simulink model "relative_dynamics_Earth_SK"  (R2021a)
settings: Solver=VariableStepAuto  StartTime=0.0  StopTime=53020  FixedStep=5  RelTol=1e-9  AbsTol=1e-11
undefined symbols (not defined in the file): a, d_lp, d_lp_sk, d_lp_z, e, init_conds, init_conds_z, K, K_z, km, M, M_z, n, n_lp, n_lp_sk, n_lp_z, r_target, s
libraries: vrlib x3, aerolibcelestial x2
settings Model: Creator=danie  LastModifiedBy=danie
settings SolverCC: AlgebraicLoopSolver=TrustRegion
settings DebuggingCC: SFMachineParentedDataDiag=warning

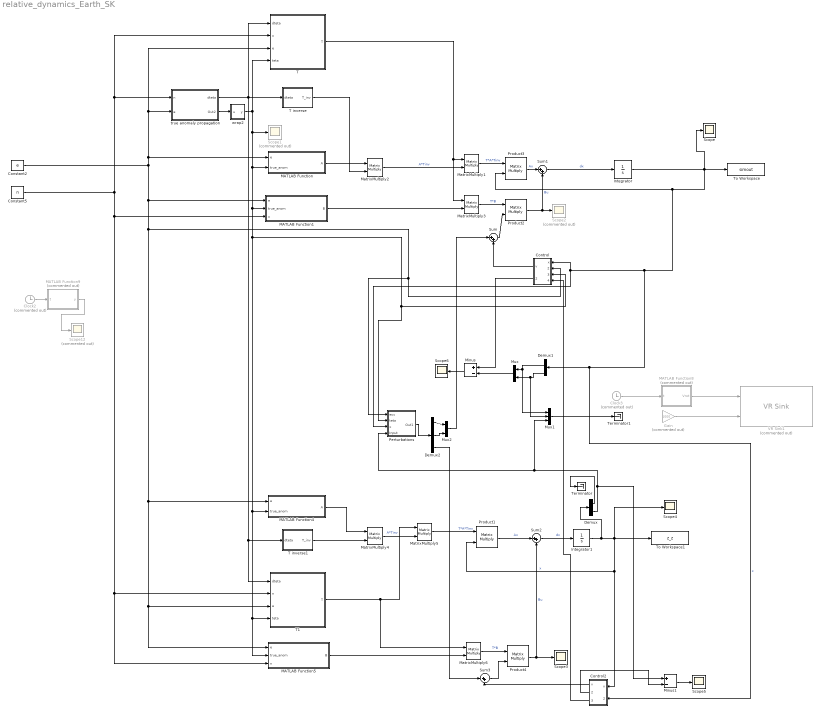
== system relative_dynamics_Earth_SK ==
  Clock2 : Clock  Commented=on
  Clock3 : Clock  Commented=on
  Constant2 : Constant  Value=e
  Constant5 : Constant  Value=n
  Control : Subsystem
  Control2 : Subsystem
  Demux : Demux  Outputs=2
  Demux1 : Demux
  Demux2 : Demux  Outputs=3
  Gain : Gain  Commented=on  Gain=1000
  Integrator : Integrator  InitialCondition=init_conds
  Integrator1 : Integrator  InitialCondition=init_conds_z
  MATLAB Function : MATLAB Function  TreatAsAtomicUnit=on
  MATLAB Function1 : MATLAB Function  TreatAsAtomicUnit=on
  MATLAB Function4 : MATLAB Function  TreatAsAtomicUnit=on
  MATLAB Function5 : MATLAB Function  TreatAsAtomicUnit=on
  MATLAB Function8 : MATLAB Function  Commented=on  TreatAsAtomicUnit=on
  MATLAB Function9 : MATLAB Function  Commented=on  TreatAsAtomicUnit=on
  MatrixMultiply{1..6} (6 alike) : Product  Multiplication=Matrix(*)
  Minus : Sum  Inputs=+-
  Minus1 : Sum  Inputs=+-
  Mux : Mux  Inputs=2
  Mux1 : Mux  Inputs=3
  Mux2 : Mux  Inputs=2
  Perturbations : Subsystem
  Product{1..4} (4 alike) : Product  SCDEnableBlockLinearizationSpecification=on  Multiplication=Matrix(*)
  Scope{,3..6} (5 alike) : Scope
  Scope1 : Scope  Commented=on
  Scope12 : Scope  Commented=on
  Scope2 : Scope  Commented=on
  Sum{,1..3} (4 alike) : Sum  Inputs=|++
  T : MATLAB Function  TreatAsAtomicUnit=on
  T inverse : MATLAB Function  TreatAsAtomicUnit=on
  T inverse1 : MATLAB Function  TreatAsAtomicUnit=on
  T1 : MATLAB Function  TreatAsAtomicUnit=on
  Terminator : Terminator
  Terminator1 : Terminator
  To Workspace : ToWorkspace  VariableName=simout  SaveFormat=Timeseries  SampleTime=-1
  To Workspace1 : ToWorkspace  VariableName=z_z  SaveFormat=Timeseries  SampleTime=-1
  VR Sink1 : vrlib/VR Sink  Commented=on  InstantiateOnLoad=on  SampleTime=0.1  ViewEnable=on  RemoteChange=off  RemoteView=off  FieldsWritten=STLEXP_Transform.rotation.4.1.1.double#node_Transform.translation.3.1.1.double  WorldFileName=try_ito.x3d  AutoView=off  VideoDimensions=[]  AllowVariableSize=off
  true anomaly propagation : Subsystem
  wrap2 : MATLAB Function  TreatAsAtomicUnit=on
  wires:
  Constant5/1 -> MATLAB Function5/3(n), T1/2(n), MATLAB Function1/3(n), T/2(n), true anomaly propagation/1(n)
  Integrator/1 -> Scope/1, To Workspace/1, Control2/2(Input), Demux1/1, Control/1(x), Perturbations/3(x), Product3/2  "x"
  Constant2/1 -> MATLAB Function5/1(e), T1/3(e), MATLAB Function4/1(e), Control/2(Input), Perturbations/1(ecc), MATLAB Function1/1(e), T/3(e), true anomaly propagation/2(e), MATLAB Function/1(e)
  Product3/1 -> Sum1/1  "Ax"
  Product2/1 -> Sum1/2, Scope2/1  "Bu"
  Sum1/1 -> Integrator/1  "dx"
  true anomaly propagation/1(dteta) -> T inverse/1(dteta), T/1(dteta), T1/1(dteta), T inverse1/1(dteta)
  true anomaly propagation/2(Out2) -> wrap2/1(u)
  T/1(T) -> MatrixMultiply3/1, MatrixMultiply1/1
  MatrixMultiply1/1 -> Product3/1  "T*A*Tinv"
  T inverse/1(T_inv) -> MatrixMultiply2/2
  MATLAB Function1/1(B) -> MatrixMultiply3/2
  MATLAB Function/1(A) -> MatrixMultiply2/1
  MatrixMultiply2/1 -> MatrixMultiply1/2  "A*Tinv"
  wrap2/1(y) -> Scope1/1, MATLAB Function5/2(true_anom), T1/4(teta), MATLAB Function4/2(true_anom), Perturbations/2(teta), Control/3(Input1), MATLAB Function1/2(true_anom), MATLAB Function/2(true_anom), T/4(teta)
  MatrixMultiply3/1 -> Product2/1  "T*B"
  T inverse1/1(T_inv) -> MatrixMultiply4/2
  MATLAB Function4/1(A) -> MatrixMultiply4/1
  MatrixMultiply4/1 -> MatrixMultiply5/2  "A*Tinv"
  T1/1(T) -> MatrixMultiply6/1, MatrixMultiply5/1
  MatrixMultiply5/1 -> Product1/1  "T*A*Tinv"
  Product1/1 -> Sum2/1  "Ax"
  Sum2/1 -> Integrator1/1  "dx"
  Integrator1/1 -> Demux/1, Scope4/1, To Workspace1/1, Product1/2, Control2/1(x)  "x"
  Product4/1 -> Scope3/1, Sum2/2  "Bu"
  MATLAB Function5/1(B) -> MatrixMultiply6/2
  MatrixMultiply6/1 -> Product4/1  "T*B"
  Sum/1 -> Product2/2
  Clock2/1 -> MATLAB Function9/1(t)
  MATLAB Function9/1(y) -> Scope12/1
  Control/1(v) -> Sum/2
  Perturbations/1(Out1) -> Demux2/1
  Demux1/2 -> Mux1/1, Mux/1
  Mux/1 -> Minus/2
  Control/2(Output) -> Minus/1
  Minus/1 -> Scope6/1
  Demux1/4 -> Mux1/2, Mux/2
  MATLAB Function8/1(Vrot) -> VR Sink1/1
  Clock3/1 -> MATLAB Function8/1(t)
  Gain/1 -> VR Sink1/2
  Demux/2 -> Minus1/1, Mux1/3, Perturbations/4(Input)
  Demux/1 -> Terminator/1
  Demux2/1 -> Mux2/1
  Demux2/2 -> Mux2/2
  Mux2/1 -> Sum/1
  Control2/1(v) -> Sum3/2
  Demux2/3 -> Sum3/1
  Sum3/1 -> Product4/2
  Control2/2(Output) -> Minus1/2
  Minus1/1 -> Scope5/1
  Control2/3(Output1) -> Control/4(Input2)
  Mux1/1 -> Terminator1/1

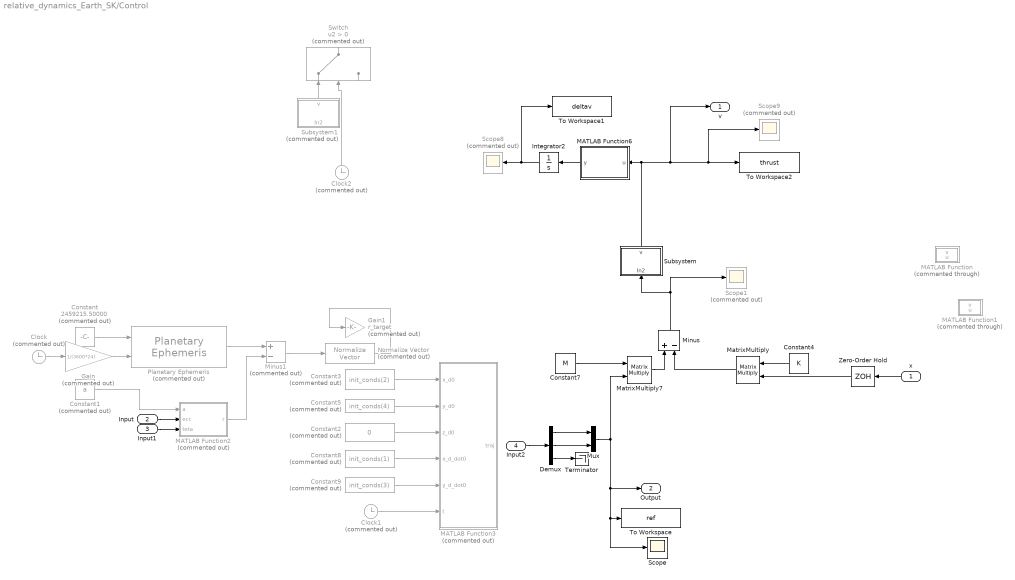
== system relative_dynamics_Earth_SK/Control ==
  x : Inport
  Input : Inport  Port=2
  Input1 : Inport  Port=3
  Input2 : Inport  Port=4
  Clock : Clock  Commented=on
  Clock1 : Clock  Commented=on
  Clock2 : Clock  Commented=on
  Constant : Constant  Commented=on  Value=2459215.50000
  Constant1 : Constant  Commented=on  Value=a
  Constant2 : Constant  Commented=on  Value=0
  Constant3 : Constant  Commented=on  Value=init_conds(2)
  Constant4 : Constant  Value=K
  Constant5 : Constant  Commented=on  Value=init_conds(4)
  Constant7 : Constant  Value=M
  Constant8 : Constant  Commented=on  Value=init_conds(1)
  Constant9 : Constant  Commented=on  Value=init_conds(3)
  Demux : Demux  Outputs=3
  Gain : Gain  Commented=on  Gain=1/(3600*24)
  Gain1 : Gain  Commented=on  Gain=r_target
  Integrator2 : Integrator
  MATLAB Function : MATLAB Function  Commented=through  TreatAsAtomicUnit=on
  MATLAB Function1 : MATLAB Function  Commented=through  TreatAsAtomicUnit=on
  MATLAB Function2 : MATLAB Function  Commented=on  TreatAsAtomicUnit=on
  MATLAB Function3 : MATLAB Function  Commented=on  TreatAsAtomicUnit=on
  MATLAB Function6 : MATLAB Function  TreatAsAtomicUnit=on
  MatrixMultiply : Product  Multiplication=Matrix(*)
  MatrixMultiply7 : Product  Multiplication=Matrix(*)
  Minus : Sum  Inputs=+-
  Minus1 : Sum  Commented=on  Inputs=+-
  Mux : Mux  Inputs=2
  Normalize Vector : vrlib/Utilities/Normalize Vector  Commented=on  maxzero=0
  Planetary Ephemeris : aerolibcelestial/Planetary Ephemeris  Commented=on  kmflag=km,km/s  epochflag=T0 and elapsed Julian time  de=DE405  nCenter=Sun  nTarget=Earth  errorflag=Error  velflag=off
      settings: SourceProductBaseCode=AE
  Scope : Scope
  Scope1 : Scope  Commented=on
  Scope8 : Scope  Commented=on
  Scope9 : Scope  Commented=on
  Subsystem : Subsystem
  Subsystem1 : Subsystem  Commented=on
  Switch : Switch  Commented=on  Criteria=u2 > Threshold
  Terminator : Terminator
  To Workspace : ToWorkspace  VariableName=ref  SaveFormat=Timeseries  SampleTime=-1
  To Workspace1 : ToWorkspace  VariableName=deltav  SaveFormat=Timeseries  SampleTime=-1
  To Workspace2 : ToWorkspace  VariableName=thrust  SaveFormat=Timeseries  SampleTime=-1
  Zero-Order Hold : ZeroOrderHold
  v : Outport
  Output : Outport  Port=2
  wires:
  Integrator2/1 -> Scope8/1, To Workspace1/1
  Constant4/1 -> MatrixMultiply/1
  MATLAB Function6/1(y) -> Integrator2/1
  MatrixMultiply7/1 -> Minus/1
  MatrixMultiply/1 -> Minus/2
  Zero-Order Hold/1 -> MatrixMultiply/2
  Constant7/1 -> MatrixMultiply7/1
  x/1 -> Zero-Order Hold/1
  Constant/1 -> Planetary Ephemeris/1
  Gain/1 -> Planetary Ephemeris/2
  Clock/1 -> Gain/1
  Constant1/1 -> MATLAB Function2/1(a)
  Input/1 -> MATLAB Function2/2(ecc)
  Input1/1 -> MATLAB Function2/3(teta)
  Planetary Ephemeris/1 -> Minus1/1
  MATLAB Function2/1(r) -> Minus1/2
  Minus1/1 -> Normalize Vector/1
  Normalize Vector/1 -> Gain1/1
  Demux/1 -> Mux/1
  Demux/2 -> Mux/2
  Demux/3 -> Terminator/1
  Mux/1 -> MatrixMultiply7/2, Scope/1, To Workspace/1, Output/1
  Minus/1 -> Subsystem/1(In2), Scope1/1
  Subsystem/1(v) -> MATLAB Function6/1(u), Scope9/1, To Workspace2/1, v/1
  Constant2/1 -> MATLAB Function3/3(z_d0)
  Constant3/1 -> MATLAB Function3/1(x_d0)
  Constant5/1 -> MATLAB Function3/2(y_d0)
  Constant8/1 -> MATLAB Function3/4(x_d_dot0)
  Constant9/1 -> MATLAB Function3/5(y_d_dot0)
  Clock1/1 -> MATLAB Function3/6(t)
  Input2/1 -> Demux/1
  Subsystem1/1(v) -> Switch/1
  Clock2/1 -> Switch/2

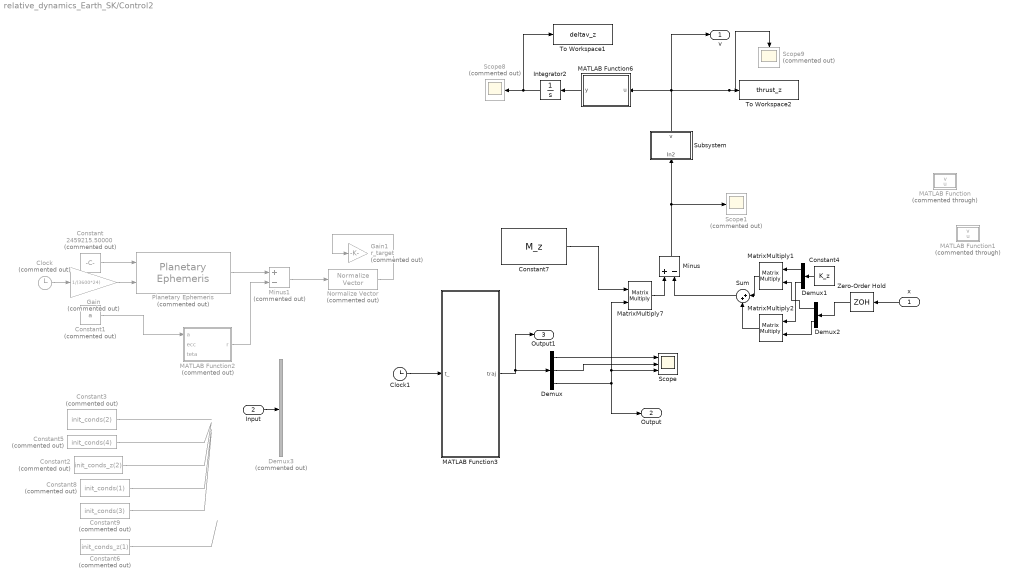
== system relative_dynamics_Earth_SK/Control2 ==
  x : Inport
  Input : Inport  Port=2
  Clock : Clock  Commented=on
  Clock1 : Clock
  Constant : Constant  Commented=on  Value=2459215.50000
  Constant1 : Constant  Commented=on  Value=a
  Constant2 : Constant  Commented=on  Value=init_conds_z(2)
  Constant3 : Constant  Commented=on  Value=init_conds(2)
  Constant4 : Constant  Value=K_z
  Constant5 : Constant  Commented=on  Value=init_conds(4)
  Constant6 : Constant  Commented=on  Value=init_conds_z(1)
  Constant7 : Constant  Value=M_z
  Constant8 : Constant  Commented=on  Value=init_conds(1)
  Constant9 : Constant  Commented=on  Value=init_conds(3)
  Demux : Demux  Outputs=3
  Demux1 : Demux  Outputs=2
  Demux2 : Demux  Outputs=2
  Demux3 : Demux  Commented=on
  Gain : Gain  Commented=on  Gain=1/(3600*24)
  Gain1 : Gain  Commented=on  Gain=r_target
  Integrator2 : Integrator
  MATLAB Function : MATLAB Function  Commented=through  TreatAsAtomicUnit=on
  MATLAB Function1 : MATLAB Function  Commented=through  TreatAsAtomicUnit=on
  MATLAB Function2 : MATLAB Function  Commented=on  TreatAsAtomicUnit=on
  MATLAB Function3 : MATLAB Function  TreatAsAtomicUnit=on
  MATLAB Function6 : MATLAB Function  TreatAsAtomicUnit=on
  MatrixMultiply1 : Product  Multiplication=Matrix(*)
  MatrixMultiply2 : Product  Multiplication=Matrix(*)
  MatrixMultiply7 : Product  Multiplication=Matrix(*)
  Minus : Sum  Inputs=+-
  Minus1 : Sum  Commented=on  Inputs=+-
  Normalize Vector : vrlib/Utilities/Normalize Vector  Commented=on  maxzero=0
  Planetary Ephemeris : aerolibcelestial/Planetary Ephemeris  Commented=on  kmflag=km,km/s  epochflag=T0 and elapsed Julian time  de=DE405  nCenter=Sun  nTarget=Earth  errorflag=Error  velflag=off
      settings: SourceProductBaseCode=AE
  Scope : Scope  NumInputPorts=3
  Scope1 : Scope  Commented=on
  Scope8 : Scope  Commented=on
  Scope9 : Scope  Commented=on
  Subsystem : Subsystem
  Sum : Sum  Inputs=|++
  To Workspace1 : ToWorkspace  VariableName=deltav_z  SaveFormat=Timeseries  SampleTime=-1
  To Workspace2 : ToWorkspace  VariableName=thrust_z  SaveFormat=Timeseries  SampleTime=-1
  Zero-Order Hold : ZeroOrderHold
  v : Outport
  Output : Outport  Port=2
  Output1 : Outport  Port=3
  wires:
  Integrator2/1 -> Scope8/1, To Workspace1/1
  MATLAB Function6/1(y) -> Integrator2/1
  MatrixMultiply7/1 -> Minus/1
  Sum/1 -> Minus/2
  Constant7/1 -> MatrixMultiply7/1
  x/1 -> Zero-Order Hold/1
  Constant/1 -> Planetary Ephemeris/1
  Gain/1 -> Planetary Ephemeris/2
  Clock/1 -> Gain/1
  Constant1/1 -> MATLAB Function2/1(a)
  Planetary Ephemeris/1 -> Minus1/1
  MATLAB Function2/1(r) -> Minus1/2
  Minus1/1 -> Normalize Vector/1
  Normalize Vector/1 -> Gain1/1
  Demux/3 -> Scope/3, MatrixMultiply7/2, Output/1
  Minus/1 -> Scope1/1, Subsystem/1(In2)
  Subsystem/1(v) -> MATLAB Function6/1(u), Scope9/1, To Workspace2/1, v/1
  MATLAB Function3/1(traj) -> Output1/1, Demux/1
  Demux/1 -> Scope/1
  Constant4/1 -> Demux1/1
  Zero-Order Hold/1 -> Demux2/1
  MatrixMultiply1/1 -> Sum/1
  MatrixMultiply2/1 -> Sum/2
  Demux1/1 -> MatrixMultiply1/1
  Demux2/1 -> MatrixMultiply1/2
  Demux1/2 -> MatrixMultiply2/1
  Demux2/2 -> MatrixMultiply2/2
  Input/1 -> Demux3/1
  Demux/2 -> Scope/2
  Clock1/1 -> MATLAB Function3/1(t_)
  Constant3/1 -> ?
  Constant5/1 -> ?
  Constant2/1 -> ?
  Constant8/1 -> ?
  Constant9/1 -> ?
  Constant6/1 -> ?

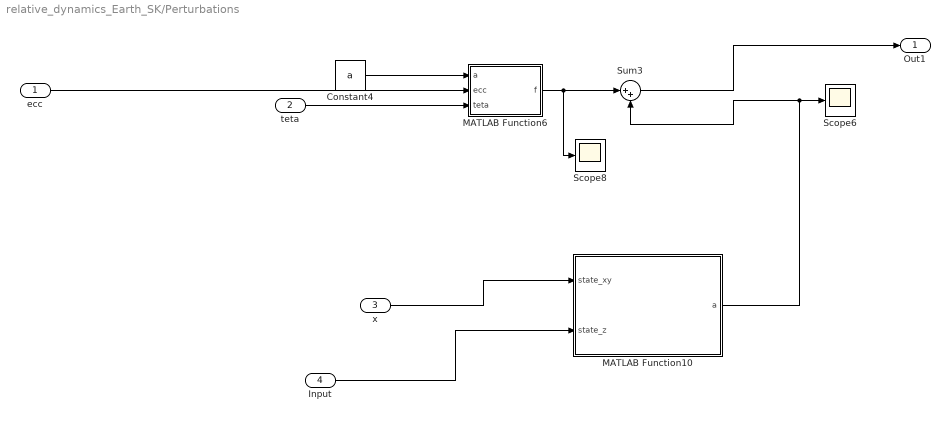
== system relative_dynamics_Earth_SK/Perturbations ==
  ecc : Inport
  teta : Inport  Port=2
  x : Inport  Port=3
  Input : Inport  Port=4
  Constant4 : Constant  Value=a
  MATLAB Function10 : MATLAB Function  TreatAsAtomicUnit=on
  MATLAB Function6 : MATLAB Function  TreatAsAtomicUnit=on
  Scope6 : Scope
  Scope8 : Scope
  Sum3 : Sum  Inputs=|++
  Out1 : Outport
  wires:
  ecc/1 -> MATLAB Function6/2(ecc)
  MATLAB Function6/1(f) -> Scope8/1, Sum3/1
  MATLAB Function10/1(a) -> Sum3/2, Scope6/1
  Constant4/1 -> MATLAB Function6/1(a)
  Sum3/1 -> Out1/1
  x/1 -> MATLAB Function10/1(state_xy)
  teta/1 -> MATLAB Function6/3(teta)
  Input/1 -> MATLAB Function10/2(state_z)

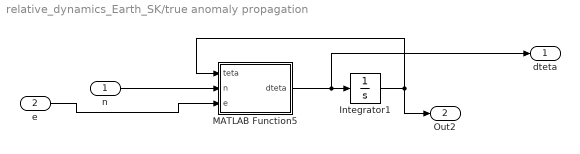
== system relative_dynamics_Earth_SK/true anomaly propagation ==
  n : Inport
  e : Inport  Port=2
  Integrator1 : Integrator
  MATLAB Function5 : MATLAB Function  TreatAsAtomicUnit=on
  dteta : Outport
  Out2 : Outport  Port=2
  wires:
  MATLAB Function5/1(dteta) -> dteta/1, Integrator1/1
  e/1 -> MATLAB Function5/3(e)
  Integrator1/1 -> Out2/1, MATLAB Function5/1(teta)
  n/1 -> MATLAB Function5/2(n)

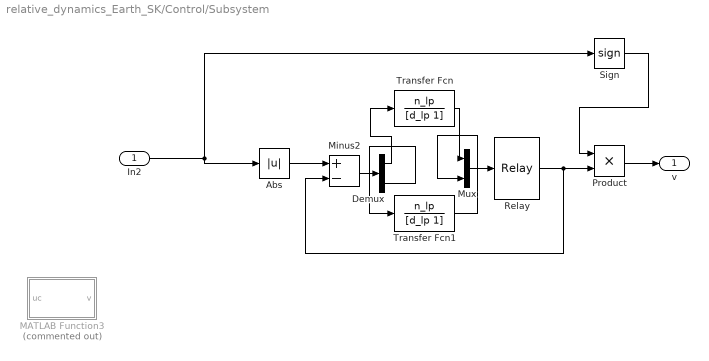
== system relative_dynamics_Earth_SK/Control/Subsystem ==
  In2 : Inport
  Abs : Abs
  Demux : Demux  Outputs=2
  MATLAB Function3 : MATLAB Function  Commented=on  TreatAsAtomicUnit=on
  Minus2 : Sum  Inputs=+-
  Mux : Mux  Inputs=2
  Product : Product
  Relay : Relay  OnSwitchValue=0.00005  OffSwitchValue=0.00000005  OnOutputValue=0.00005
  Sign : Signum
  Transfer Fcn : TransferFcn  Numerator=n_lp  Denominator=[d_lp 1]
  Transfer Fcn1 : TransferFcn  Numerator=n_lp  Denominator=[d_lp 1]
  v : Outport
  wires:
  Relay/1 -> Product/2, Minus2/2
  Abs/1 -> Minus2/1
  In2/1 -> Sign/1, Abs/1
  Mux/1 -> Relay/1
  Product/1 -> v/1
  Sign/1 -> Product/1
  Minus2/1 -> Demux/1
  Demux/1 -> Transfer Fcn/1
  Demux/2 -> Transfer Fcn1/1
  Transfer Fcn/1 -> Mux/1
  Transfer Fcn1/1 -> Mux/2

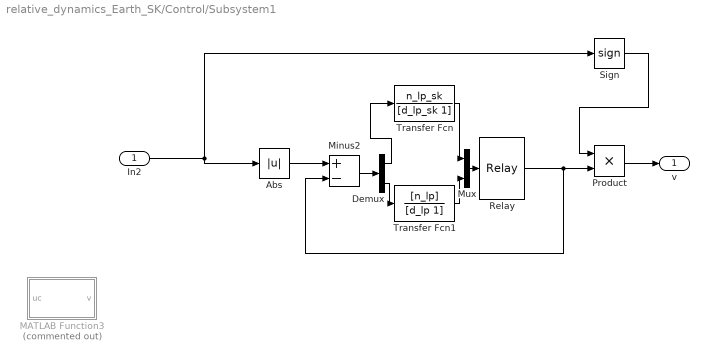
== system relative_dynamics_Earth_SK/Control/Subsystem1 ==
  In2 : Inport
  Abs : Abs
  Demux : Demux  Outputs=2
  MATLAB Function3 : MATLAB Function  Commented=on  TreatAsAtomicUnit=on
  Minus2 : Sum  Inputs=+-
  Mux : Mux  Inputs=2
  Product : Product
  Relay : Relay  OnSwitchValue=0.00001  OffSwitchValue=0.0000001  OnOutputValue=0.00001
  Sign : Signum
  Transfer Fcn : TransferFcn  Numerator=n_lp_sk  Denominator=[d_lp_sk 1]
  Transfer Fcn1 : TransferFcn  Numerator=[n_lp]  Denominator=[d_lp 1]
  v : Outport
  wires:
  Relay/1 -> Product/2, Minus2/2
  Abs/1 -> Minus2/1
  In2/1 -> Sign/1, Abs/1
  Mux/1 -> Relay/1
  Product/1 -> v/1
  Sign/1 -> Product/1
  Minus2/1 -> Demux/1
  Demux/1 -> Transfer Fcn/1
  Demux/2 -> Transfer Fcn1/1
  Transfer Fcn/1 -> Mux/1
  Transfer Fcn1/1 -> Mux/2

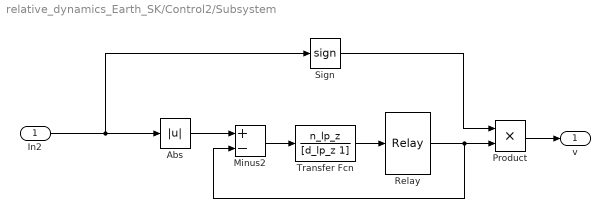
== system relative_dynamics_Earth_SK/Control2/Subsystem ==
  In2 : Inport
  Abs : Abs
  Minus2 : Sum  Inputs=+-
  Product : Product
  Relay : Relay  OnSwitchValue=0.000005  OffSwitchValue=0.00000005  OnOutputValue=0.000005
  Sign : Signum
  Transfer Fcn : TransferFcn  Numerator=n_lp_z  Denominator=[d_lp_z 1]
  v : Outport
  wires:
  Relay/1 -> Product/2, Minus2/2
  Abs/1 -> Minus2/1
  In2/1 -> Sign/1, Abs/1
  Transfer Fcn/1 -> Relay/1
  Product/1 -> v/1
  Sign/1 -> Product/1
  Minus2/1 -> Transfer Fcn/1

== matlab function relative_dynamics_Earth_SK/Control/MATLAB Function6 ==
  data: u input; y output
function y = fcn(u)

y =norm(u);

== matlab function relative_dynamics_Earth_SK/Control2/MATLAB Function ==
  data: u input; v output
function v = fcn(u)
v=[0;0];
if abs(u(1))>0.00001
    v(1)=sign(u(1))*0.00001;
else
    v(1)=u(1);
end
if abs(u(2))>0.00001
    v(2)=sign(u(2))*0.00001;
else
    v(2)=u(2);
end

== matlab function relative_dynamics_Earth_SK/Perturbations/MATLAB Function6 ==
  data: a input; f output; ecc input; teta input
function f = SRP(a,ecc,teta)
S=1358.0; %W/m2
AU=149597870.0; %km
Cr=1.4;
m=100;%kg
A=10;%m^2
c=299792458; %m/s
r=a*(1-(ecc^2))/(1+ecc*cos(teta));
f=S*(AU^2)*Cr*A/(m*(r^2)*c)*[1;0;0]; %m/s
f=f/1000;

== matlab function relative_dynamics_Earth_SK/MATLAB Function9 ==
  data: t input; y output
function y = fcn(t)
if t<=5
    %f is m/s^2, assuming 100kg mass this is 1N, ok for ramp
    y=[-21+0.5*0.001*(t^2) 0]';
elseif and(t>=5,t<=10)
    y=[-21+0.025-0.5*0.001*(t^2) 0]';
else
    y=[-21 0]';
end

== matlab function relative_dynamics_Earth_SK/Perturbations/MATLAB Function10 ==
  data: state_xy input; a output; state_z input
function a  = asteroid_gravity_point_model(state_xy,state_z)
G=6.674e-11; %m3/(kg*s2)
mass= 2.090805433926013e+08;%kg%Bennu
mu=mass*G;
r_=[state_xy(2),state_xy(4),state_z].*1000;
r=norm(r_);
a=((-mu*r_/(r^3))/1000)'; %km/s^2

== matlab function relative_dynamics_Earth_SK/Control/MATLAB Function ==
  data: u input; v output
function v = fcn(u)
v=[0;0];
if abs(u(1))>0.00001
    v(1)=sign(u(1))*0.00001;
else
    v(1)=u(1);
end
if abs(u(2))>0.00001
    v(2)=sign(u(2))*0.00001;
else
    v(2)=u(2);
end

== matlab function relative_dynamics_Earth_SK/MATLAB Function1 ==
  data: e input; B output; true_anom input; n input
function B = B_ss(e,true_anom,n)
B=((1-(e^2))^3)/(((1+e*cos(true_anom))^4)*(n^2))*[1 0; 0 0; 0 1; 0 0];

== matlab function relative_dynamics_Earth_SK/Control/MATLAB Function1 ==
  data: u input; v output
function v = fcn(u)
v=[0;0];
if abs(u(1))<0.000001
    v(1)=0;
else
    v(1)=u(1);
end
if abs(u(2))<0.000001
    v(2)=0;
else
    v(2)=u(2);
end

== matlab function relative_dynamics_Earth_SK/Control/MATLAB Function2 ==
  data: a input; ecc input; r output; teta input
function r = fcn(a,ecc,teta)
R=a*(1-(ecc^2))/(1+ecc*cos(teta));
x=R*cos(teta);
y=R*sin(teta);
r=[x,y,0];

== matlab function relative_dynamics_Earth_SK/Control/Subsystem/MATLAB Function3 ==
  data: uc input; v output
function v = fcn(uc)
v=[0;0];
uon=0.0001;
uthrust=0.000001;
uoff=0.0000009;
if abs(uc(1))>=uoff%,abs(uc(1))<=uon)
    v(1)=sign(uc(1))*uthrust;
else
    v(1)=0;
end
if abs(uc(2))>=uoff
    v(2)=sign(uc(2))*uthrust;
else
    v(2)=0;
end

== matlab function relative_dynamics_Earth_SK/Control/MATLAB Function3 ==
  data: traj output; x_d0 input; y_d0 input; z_d0 input; x_d_dot0 input; y_d_dot0 input; t input
function traj  = fcn(x_d0,y_d0,z_d0,x_d_dot0,y_d_dot0,t)
% x_d0=50;
% =0;
% y_d0=50;
% =0;
% z_d0=2000;
z_d_dot0=0;
tao=20000;
traj=zeros(3,1);
traj(1)=(x_d_dot0*tao+2*x_d0)*t^3/tao^3 - (2*x_d_dot0*tao+3*x_d0)*t^2/tao^2 + x_d_dot0*t + x_d0;
traj(2)=(y_d_dot0*tao+2*y_d0)*t^3/tao^3 - (2*y_d_dot0*tao+3*y_d0)*t^2/tao^2 + y_d_dot0*t + y_d0;
traj(3)=(z_d_dot0*tao+2*z_d0)*t^3/tao^3 - (2*z_d_dot0*tao+3*z_d0)*t^2/tao^2 + z_d_dot0*t + z_d0;
end

== matlab function relative_dynamics_Earth_SK/MATLAB Function8 ==
  data: t input; Vrot output
function Vrot = fcn(t)
w=2*pi/250;
Vrot=[sqrt(2) sqrt(2) 0 w*t];

== matlab function relative_dynamics_Earth_SK/Control2/MATLAB Function1 ==
  data: u input; v output
function v = fcn(u)
v=[0;0];
if abs(u(1))<0.000001
    v(1)=0;
else
    v(1)=u(1);
end
if abs(u(2))<0.000001
    v(2)=0;
else
    v(2)=u(2);
end

== matlab function relative_dynamics_Earth_SK/Control2/MATLAB Function2 ==
  data: a input; ecc input; r output; teta input
function r = fcn(a,ecc,teta)
R=a*(1-(ecc^2))/(1+ecc*cos(teta));
x=R*cos(teta);
y=R*sin(teta);
r=[x,y,0];

== matlab function relative_dynamics_Earth_SK/Control2/MATLAB Function3 ==
  data: traj output; t_ input
function traj  = fcn(t_)
% x_d0=50;
% =0;
% y_d0=50;
% =0;
% z_d0=2000;
% z_d_dot0=0;
r_ast=0.0431/2;%km
traj=zeros(3,1);
x_d_dot0=0;
y_d_dot0=0;
z_d_dot0=0;
% OPERATION STRUCTURE %
sk_2000_time=30*3600; %1 hours sk 
descent_200_time=5*3600; %5 hours initial descent
sk_200_time=40*60; %40 min
descent_10_time=1900; %31.6667 min
sk_10_time=2*60; %2 min
flyaway_time= 5.5*3600; %5.5 hours
% perturbed
perturbed=1;
if not(perturbed)
if t_<=(sk_2000_time)
    traj=[-2; 0; 0];
elseif t_<=(sk_2000_time+descent_200_time)
    tao=descent_200_time;
    t=t_-(sk_2000_time);
    final_point=[-(0.2+r_ast); 0; 0];
    x_d0=-2;
    y_d0=0;
    z_d0=0;
    x_d0_s=x_d0-final_point(1);
    y_d0_s=y_d0-final_point(2);
    z_d0_s=z_d0-final_point(3);
    traj(1)=(x_d_dot0*tao+2*x_d0_s)*t^3/tao^3 - (2*x_d_dot0*tao+3*x_d0_s)*t^2/tao^2 + x_d_dot0*t + x_d0_s + final_point(1);
    traj(2)=(y_d_dot0*tao+2*y_d0_s)*t^3/tao^3 - (2*y_d_dot0*tao+3*y_d0_s)*t^2/tao^2 + y_d_dot0*t + y_d0_s + final_point(2);
    traj(3)=(z_d_dot0*tao+2*z_d0_s)*t^3/tao^3 - (2*z_d_dot0*tao+3*z_d0_s)*t^2/tao^2 + z_d_dot0*t + z_d0_s + final_point(3);
elseif t_<=(sk_2000_time+descent_200_time+sk_200_time)
    traj=[-(0.2+r_ast); 0; 0];
elseif t_<=(sk_2000_time+descent_200_time+sk_200_time+descent_10_time)
    tao=descent_10_time;
    t=t_-(sk_2000_time+descent_200_time+sk_200_time);
    final_point=[-(0.010+r_ast); 0; 0];
    x_d0=-(0.2+r_ast);
    y_d0=0;
    z_d0=0;
    x_d0_s=x_d0-final_point(1);
    y_d0_s=y_d0-final_point(2);
    z_d0_s=z_d0-final_point(3);
    traj(1)=(x_d_dot0*tao+2*x_d0_s)*t^3/tao^3 - (2*x_d_dot0*tao+3*x_d0_s)*t^2/tao^2 + x_d_dot0*t + x_d0_s + final_point(1);
    traj(2)=(y_d_dot0*tao+2*y_d0_s)*t^3/tao^3 - (2*y_d_dot0*tao+3*y_d0_s)*t^2/tao^2 + y_d_dot0*t + y_d0_s + final_point(2);
    traj(3)=(z_d_dot0*tao+2*z_d0_s)*t^3/tao^3 - (2*z_d_dot0*tao+3*z_d0_s)*t^2/tao^2 + z_d_dot0*t + z_d0_s + final_point(3);
elseif t_<=(sk_2000_time+descent_200_time+sk_200_time+descent_10_time+sk_10_time)
    traj=[-(0.010+r_ast); 0; 0];
elseif t_<=(sk_2000_time+descent_200_time+sk_200_time+descent_10_time+sk_10_time+flyaway_time)
    tao=flyaway_time;
    t=t_-(sk_2000_time+descent_200_time+sk_200_time+descent_10_time+sk_10_time);
    final_point=[-2; 0; 0];
    x_d0=-(0.010+r_ast);
    y_d0=0;
    z_d0=0;
    x_d0_s=x_d0-final_point(1);
    y_d0_s=y_d0-final_point(2);
    z_d0_s=z_d0-final_point(3);
    traj(1)=(x_d_dot0*tao+2*x_d0_s)*t^3/tao^3 - (2*x_d_dot0*tao+3*x_d0_s)*t^2/tao^2 + x_d_dot0*t + x_d0_s + final_point(1);
    traj(2)=(y_d_dot0*tao+2*y_d0_s)*t^3/tao^3 - (2*y_d_dot0*tao+3*y_d0_s)*t^2/tao^2 + y_d_dot0*t + y_d0_s + final_point(2);
    traj(3)=(z_d_dot0*tao+2*z_d0_s)*t^3/tao^3 - (2*z_d_dot0*tao+3*z_d0_s)*t^2/tao^2 + z_d_dot0*t + z_d0_s + final_point(3);
end
else
    x_d_dot0=0;
    y_d_dot0=0;%.0001/sqrt(3);
    z_d_dot0=0;%.0001/sqrt(3);
    if t_<=(sk_2000_time)
    traj=[-2; 0; 0];
    elseif t_<=(sk_2000_time+descent_200_time)
    tao=descent_200_time;
    t=t_-(sk_2000_time);
    final_point=[-(0.2+r_ast); 0; 0];
    x_d0=-2;
    y_d0=0;
    z_d0=0;
    x_d0_s=x_d0-final_point(1);
    y_d0_s=y_d0-final_point(2);
    z_d0_s=z_d0-final_point(3);
    traj(1)=(x_d_dot0*tao+2*x_d0_s)*t^3/tao^3 - (2*x_d_dot0*tao+3*x_d0_s)*t^2/tao^2 + x_d_dot0*t + x_d0_s + final_point(1);
    traj(2)=(y_d_dot0*tao+2*y_d0_s)*t^3/tao^3 - (2*y_d_dot0*tao+3*y_d0_s)*t^2/tao^2 + y_d_dot0*t + y_d0_s + final_point(2);
    traj(3)=(z_d_dot0*tao+2*z_d0_s)*t^3/tao^3 - (2*z_d_dot0*tao+3*z_d0_s)*t^2/tao^2 + z_d_dot0*t + z_d0_s + final_point(3);
    elseif t_<=(sk_2000_time+descent_200_time+sk_200_time)
    traj=[-(0.2+r_ast); 0; 0];
    elseif t_<=(sk_2000_time+descent_200_time+sk_200_time+descent_10_time)
    tao=descent_10_time;
    t=t_-(sk_2000_time+descent_200_time+sk_200_time);
    final_point=[-(0.010+r_ast); 0; 0];
    x_d0=-(0.2+r_ast);
    y_d0=0;
    z_d0=0;
    x_d0_s=x_d0-final_point(1);
    y_d0_s=y_d0-final_point(2);
    z_d0_s=z_d0-final_point(3);
    traj(1)=(x_d_dot0*tao+2*x_d0_s)*t^3/tao^3 - (2*x_d_dot0*tao+3*x_d0_s)*t^2/tao^2 + x_d_dot0*t + x_d0_s + final_point(1);
    traj(2)=(y_d_dot0*tao+2*y_d0_s)*t^3/tao^3 - (2*y_d_dot0*tao+3*y_d0_s)*t^2/tao^2 + y_d_dot0*t + y_d0_s + final_point(2);
    traj(3)=(z_d_dot0*tao+2*z_d0_s)*t^3/tao^3 - (2*z_d_dot0*tao+3*z_d0_s)*t^2/tao^2 + z_d_dot0*t + z_d0_s + final_point(3);
    elseif t_<=(sk_2000_time+descent_200_time+sk_200_time+descent_10_time+sk_10_time)
    traj=[-(0.010+r_ast); 0; 0];
    elseif t_<=(sk_2000_time+descent_200_time+sk_200_time+descent_10_time+sk_10_time+flyaway_time)
    tao=flyaway_time;
    t=t_-(sk_2000_time+descent_200_time+sk_200_time+descent_10_time+sk_10_time);
    final_point=[-2; 0; 0];
    x_d0=-(0.010+r_ast);
    y_d0=0;
    z_d0=0;
    x_d0_s=x_d0-final_point(1);
    y_d0_s=y_d0-final_point(2);
    z_d0_s=z_d0-final_point(3);
    traj(1)=(x_d_dot0*tao+2*x_d0_s)*t^3/tao^3 - (2*x_d_dot0*tao+3*x_d0_s)*t^2/tao^2 + x_d_dot0*t + x_d0_s + final_point(1);
    traj(2)=(y_d_dot0*tao+2*y_d0_s)*t^3/tao^3 - (2*y_d_dot0*tao+3*y_d0_s)*t^2/tao^2 + y_d_dot0*t + y_d0_s + final_point(2);
    traj(3)=(z_d_dot0*tao+2*z_d0_s)*t^3/tao^3 - (2*z_d_dot0*tao+3*z_d0_s)*t^2/tao^2 + z_d_dot0*t + z_d0_s + final_point(3);
    end
end

== matlab function relative_dynamics_Earth_SK/Control2/MATLAB Function6 ==
  data: u input; y output
function y = fcn(u)

y =norm(u);

== matlab function relative_dynamics_Earth_SK/MATLAB Function ==
  data: e input; A output; true_anom input
function A = A_ss(e,true_anom)
A=[ 2*e*sin(true_anom)/(1+e*cos(true_anom)), (3+e*cos(true_anom))/(1+e*cos(true_anom)), 2, -2*e*sin(true_anom)/(1+e*cos(true_anom)); 
    1, 0, 0, 0;
   -2, 2*e*sin(true_anom)/(1+e*cos(true_anom)), 2*e*sin(true_anom)/(1+e*cos(true_anom)), e*cos(true_anom)/(1+e*cos(true_anom));
   0, 0, 1, 0];

== matlab function relative_dynamics_Earth_SK/Control/Subsystem1/MATLAB Function3 ==
  data: uc input; v output
function v = fcn(uc)
v=[0;0];
uon=0.0001;
uthrust=0.000001;
uoff=0.0000009;
if abs(uc(1))>=uoff%,abs(uc(1))<=uon)
    v(1)=sign(uc(1))*uthrust;
else
    v(1)=0;
end
if abs(uc(2))>=uoff
    v(2)=sign(uc(2))*uthrust;
else
    v(2)=0;
end

== matlab function relative_dynamics_Earth_SK/T ==
  data: dteta input; T output; n input; e input; teta input
function T = fcn(dteta, n,e,teta)
T=[dteta^2 dteta*(-(n*2*(1+e*cos(teta))*e*sin(teta)/((1-e^2)^1.5))) 0 0; 0 dteta 0 0; 0 0 dteta^2 dteta*(-(n*2*(1+e*cos(teta))*e*sin(teta)/((1-e^2)^1.5))); 0 0 0 dteta];

== matlab function relative_dynamics_Earth_SK/true anomaly propagation/MATLAB Function5 ==
  data: teta input; n input; dteta output; e input
function dteta = fcn(teta,n,e)
dteta=(n*(1+e*cos(teta))^2)/((1-e^2)^1.5);

== matlab function relative_dynamics_Earth_SK/wrap2 ==
  data: u input; y output
function y = fcn(u)

y = mod(u,2*pi);

== matlab function relative_dynamics_Earth_SK/T inverse ==
  data: dteta input; T_inv output
function T_inv = fcn(dteta)
T_inv=[1/dteta 0 0 0; 0 1 0 0; 0 0 1/dteta 0; 0 0 0 1];

== matlab function relative_dynamics_Earth_SK/MATLAB Function4 ==
  data: e input; A output; true_anom input
function A = A_ss_z(e,true_anom)
A=[2*e*sin(true_anom)/(1+e*cos(true_anom)) -1/(1+e*cos(true_anom)); 1 0];

== matlab function relative_dynamics_Earth_SK/T inverse1 ==
  data: dteta input; T_inv output
function T_inv = fcn(dteta)
T_inv=[1/dteta 0; 0 1;];

== matlab function relative_dynamics_Earth_SK/T1 ==
  data: dteta input; T output; n input; e input; teta input
function T = fcn(dteta, n,e,teta)
T=[dteta^2 dteta*(-(n*2*(1+e*cos(teta))*e*sin(teta)/((1-e^2)^1.5))); 0 dteta];

== matlab function relative_dynamics_Earth_SK/MATLAB Function5 ==
  data: e input; B output; true_anom input; n input
function B = B_ss(e,true_anom,n)
B=((1-(e^2))^3)/(((1+e*cos(true_anom))^4)*(n^2))*[1; 0];
